simulink model "Backstepping"  (R2016b)
settings: Solver=ode45  StartTime=0.0  StopTime=10  RelTol=1e-5  EnableMultiTasking=on
values from neighbouring files (symbols this model uses):
  K = 3    [Plot.m]
  x0 = [0 0 0.1]    [Plot.m]
  x0_hat = [8.3, 6.2, -14.5]    [Plot.m]
settings Model: Creator=Emanuele  LastModifiedBy=danielesmn
settings DataIOCC: LimitDataPoints=on  SaveFormat=Array
settings OptimizationCC: LifeSpan=inf
settings DebuggingCC: UnderspecifiedInitializationDetection=Classic  MergeDetectMultiDrivingBlocksExec=none  SFUnexpectedBacktrackingDiag=warning  SFNoUnconditionalDefaultTransitionDiag=warning  SFExecutionAtInitializationDiag=none
settings HardwareCC: ProdBitPerPointer=32  ProdBitPerSizeT=32  ProdBitPerPtrDiffT=32  ProdLargestAtomicFloat=None  ProdIntDivRoundTo=Undefined  ProdEndianess=Unspecified  ProdWordSize=32  ProdHWDeviceType=32-bit Generic
settings ModelReferenceCC: PropagateSignalLabelsOutOfModel=off
settings GRTTargetCC: TargetLangStandard=C89/C90 (ANSI)  GeneratePreprocessorConditionals=Disable all
settings ConfigComp: CovMetricSettings=dw  CovHtmlReporting=on  CovSaveCumulativeToWorkspaceVar=on  CovSaveSingleToWorkspaceVar=on  CovExternalEMLEnable=off

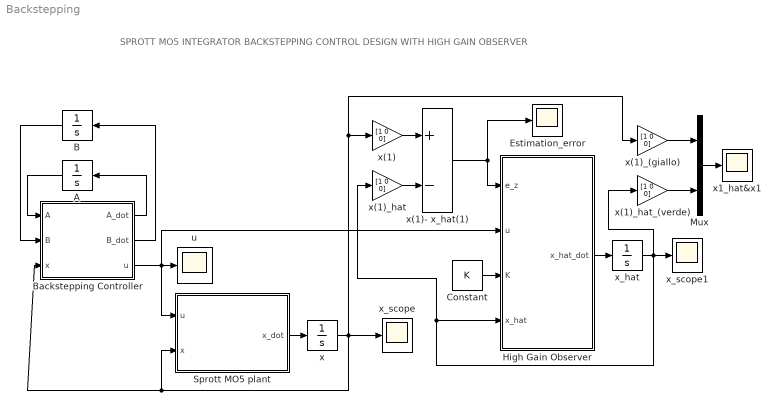
== system Backstepping ==
  note: SPROTT MO5 INTEGRATOR BACKSTEPPING CONTROL DESIGN WITH HIGH GAIN OBSERVER
  " x_scope" : Scope
  " x_scope1" : Scope
  A : Integrator  InitialCondition=15.7
  B : Integrator  InitialCondition=5.9
  Backstepping Controller : MATLAB Function  TreatAsAtomicUnit=on
  Constant : Constant  Value=K
  Estimation_error : Scope
  High Gain Observer : MATLAB Function  TreatAsAtomicUnit=on
  Mux : Mux  Inputs=2
  Sprott MO5 plant : MATLAB Function  TreatAsAtomicUnit=on
  u : Scope
  x : Integrator  InitialCondition=x0
  x(1) : Gain  Gain=[1 0 0]
  x(1)- x_hat(1) : Sum  Inputs=+-
  x(1)_(giallo) : Gain  Gain=[1 0 0]
  x(1)_hat : Gain  Gain=[1 0 0]
  x(1)_hat_(verde) : Gain  Gain=[1 0 0]
  x1_hat&x1 : Scope
  x_hat : Integrator  InitialCondition=x0_hat
  wires:
  High Gain Observer/1(x_hat_dot) -> x_hat/1
  Constant/1 -> High Gain Observer/3(K)
  Backstepping Controller/3(u) -> Sprott MO5 plant/1(u), High Gain Observer/2(u), u/1
  Sprott MO5 plant/1(x_dot) -> x/1
  x/1 -> Sprott MO5 plant/2(x), Backstepping Controller/3(x), x(1)_(giallo)/1, x(1)/1, " x_scope"/1
  A/1 -> Backstepping Controller/1(A)
  Backstepping Controller/1(A_dot) -> A/1
  Backstepping Controller/2(B_dot) -> B/1
  B/1 -> Backstepping Controller/2(B)
  x_hat/1 -> " x_scope1"/1, High Gain Observer/4(x_hat), x(1)_hat/1, x(1)_hat_(verde)/1
  x(1)/1 -> x(1)- x_hat(1)/1
  x(1)- x_hat(1)/1 -> Estimation_error/1, High Gain Observer/1(e_z)
  x(1)_hat/1 -> x(1)- x_hat(1)/2
  Mux/1 -> x1_hat&x1/1
  x(1)_(giallo)/1 -> Mux/1
  x(1)_hat_(verde)/1 -> Mux/2

== matlab function Backstepping/Backstepping Controller ==
  data: A_dot output; B_dot output; A input; B input; u output; x input
function [A_dot, B_dot, u] = fcn(A, B, x)

Ts = 0.005;
k = 10;
eta_z = 2*x(1) + 2*x(2) + x(3);

A_dot = -x(3)*eta_z;
B_dot = -x(2)*eta_z;

%u = -4*x(1) - (5-B)*x(2) - (3-A)*x(3) + x(1)^3 -k*eta_z;

u = x(1)*(-2-2*k)+x(2)*(-3+1-2*k)+x(3)*(-2+0.7-k)+(x(3)^2)*x(1)+4*(x(1)^2)*x(3)+4*x(1)*(x(2)^2)+4*(x(1)^3)+4*x(1)*x(2)*x(3);

== matlab function Backstepping/Sprott MO5 plant ==
  data: u input; x input; x_dot output
function x_dot = Sprott_MO(u,x)

x1_dot = x(2);
x2_dot = x(3);
x3_dot = -0.7*x(3) - 1*x(2) + x(1) - x(1)^3 + u;

x_dot = [x1_dot, x2_dot, x3_dot]';

== matlab function Backstepping/High Gain Observer ==
  data: e_z input; u input; K input; x_hat input; x_hat_dot output
function x_hat_dot = HGObs(e_z, u, K, x_hat)

x = x_hat;

% Defining parameters
c0 = 7;
c1 = 8;
c2 = 9;

% High-Gain Observer
x1_hat_dot = x_hat(2) + c2*K*e_z(1);
x2_hat_dot = x_hat(3) + c1*K^2*e_z(1);
x3_hat_dot = -0.7*x_hat(3) - 1*x_hat(2) + x_hat(1) - x_hat(1)^3 + u + c0*K^3*e_z(1);

x_hat_dot = [x1_hat_dot, x2_hat_dot, x3_hat_dot]';
